simulink model "quadABLwind"  (R2018a)
settings: Solver=FixedStepAuto  StartTime=0.0  StopTime=50  FixedStep=.001  RelTol=1e-3  EnableMultiTasking=on
InitFcn:
  | parameters
model workspace: external: MAT-File C:\Users\Lab\Documents\MATLAB\projects\feedback_Ziegler_Quadrotor\parameters.mat (data not in the file)
values from neighbouring files (symbols this model uses):
  des_Position = zeros(10005/Ts + 1, 7)    [ABL_Quad_Traj.m]    (also in skyline_Quad_Traj.m = zeros(5005/Ts + 1, 7))
  wind_and_Max_Vel = abs([0, crosswind, maxVel])    [ABL_Quad_Traj.m]    (also in skyline_Quad_Traj.m)
  windECombined = [windE1; windE2; windE3; windE4; windE5; windE6; windE7]    [ABL_Quad_Traj.m]
  windNCombined = [windN1; windN2; windN3; windN4; windN5; windN6; windN7]    [ABL_Quad_Traj.m]
undefined symbols (not defined in the file or in its folder): DiscIntNeverNeededParam, P, starting_Point
libraries: simulink x1
settings Model: Creator=Lab  LastModifiedBy=lab
settings DataIOCC: ExternalInput=P
settings OptimizationCC: LifeSpan=inf
settings DebuggingCC: MultiTaskRateTransMsg=warning  SFUnexpectedBacktrackingDiag=warning  SFNoUnconditionalDefaultTransitionDiag=warning  SFExecutionAtInitializationDiag=none
settings CodeAppCC: StateflowObjectComments=on
settings GRTTargetCC: TargetLangStandard=C89/C90 (ANSI)  GeneratePreprocessorConditionals=Disable all
settings ConfigComp: CovMetricSettings=dw  CovHtmlReporting=on  CovSaveCumulativeToWorkspaceVar=on  CovSaveSingleToWorkspaceVar=on  CovExternalEMLEnable=off

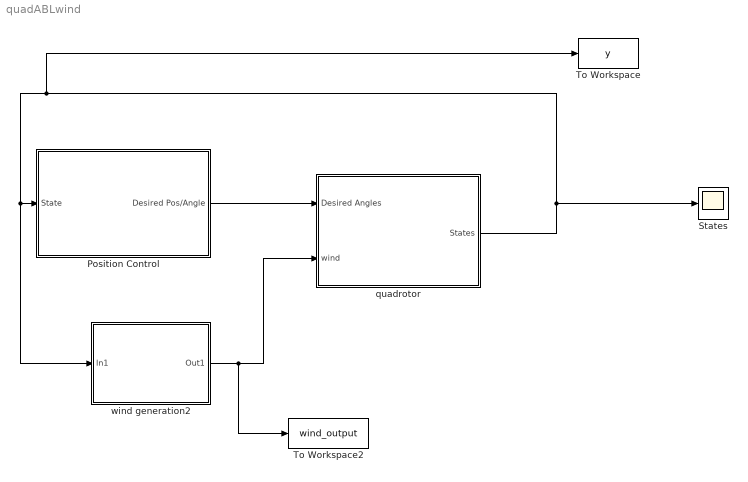
== system quadABLwind ==
  Position Control : Subsystem
  States : Scope
  To Workspace : ToWorkspace  VariableName=y  SaveFormat=Timeseries  SampleTime=-1
  To Workspace2 : ToWorkspace  VariableName=wind_output  SaveFormat=Timeseries  SampleTime=-1
  quadrotor : Subsystem
  wind generation2 : Subsystem
  wires:
  Position Control/1(Desired Pos/Angle) -> quadrotor/1(Desired Angles)
  wind generation2/1(Out1) -> To Workspace2/1, quadrotor/2(wind)
  quadrotor/1(States) -> To Workspace/1, wind generation2/1(In1), Position Control/1(State), States/1

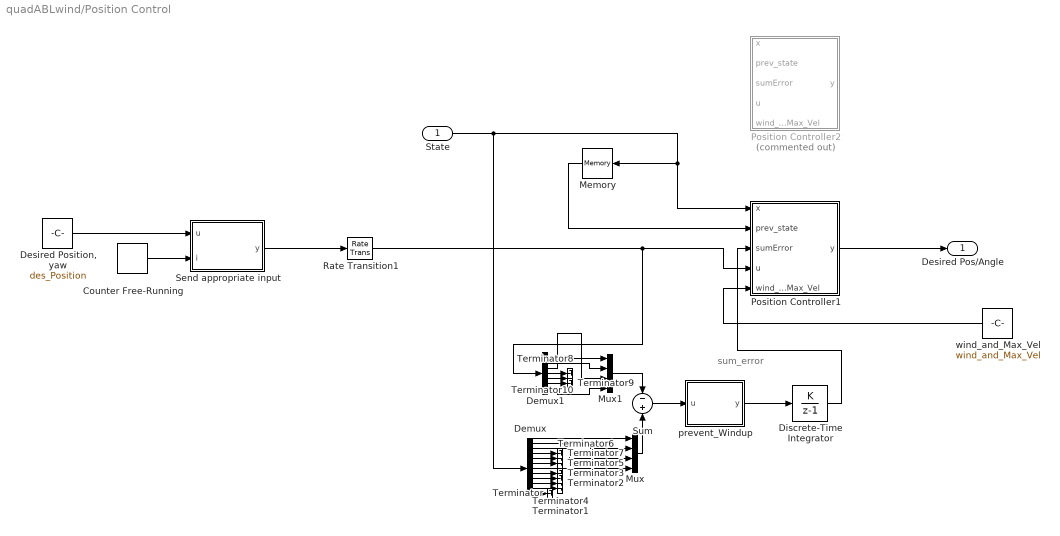
== system quadABLwind/Position Control ==
  note: sum_error
  State : Inport
  Counter Free-Running : simulink/Sources/Counter Free-Running  NumBits=32  tsamp=Ts
  Demux : Demux  Outputs=12
  Demux1 : Demux  Outputs=7
  "Desired Position, yaw" : Constant  Value=des_Position
  Discrete-Time Integrator : DiscreteIntegrator  IntegratorMethod=Accumulation: Forward Euler  gainval=1  SampleTime=-1  ICPrevOutput=DiscIntNeverNeededParam  ICPrevScaledInput=DiscIntNeverNeededParam
  Memory : Memory  InitialCondition=[0 0 0 0 0 0 0 0 0 0 0 0]
  Mux : Mux
  Mux1 : Mux
  Position Controller1 : MATLAB Function  TreatAsAtomicUnit=on  SystemSampleTime=P.Ts
  Position Controller2 : MATLAB Function  Commented=on  TreatAsAtomicUnit=on  SystemSampleTime=P.Ts
  Rate Transition1 : RateTransition  OutPortSampleTime=Tsd
  Send appropriate input : MATLAB Function  TreatAsAtomicUnit=on
  Sum : Sum  Inputs=-+
  Terminator{,1..10} (11 alike) : Terminator
  prevent_Windup : MATLAB Function  TreatAsAtomicUnit=on
  wind_and_Max_Vel : Constant  Value=wind_and_Max_Vel
  Desired Pos/Angle : Outport
  wires:
  Position Controller1/1(y) -> Desired Pos/Angle/1
  Mux/1 -> Sum/2
  Demux/1 -> Mux/1
  Demux/2 -> Mux/2
  Demux/3 -> Mux/3
  Memory/1 -> Position Controller1/2(prev_state)
  Sum/1 -> prevent_Windup/1(u)
  Demux/7 -> Mux/4
  "Desired Position, yaw"/1 -> Send appropriate input/1(u)
  Counter Free-Running/1 -> Send appropriate input/2(i)
  Send appropriate input/1(y) -> Rate Transition1/1
  State/1 -> Demux/1, Position Controller1/1(x), Memory/1
  Rate Transition1/1 -> Position Controller1/4(u), Demux1/1
  wind_and_Max_Vel/1 -> Position Controller1/5(wind_and_Max_Vel)
  Discrete-Time Integrator/1 -> Position Controller1/3(sumError)
  Demux1/1 -> Mux1/1
  Demux1/2 -> Mux1/2
  Demux1/3 -> Mux1/3
  Demux1/7 -> Mux1/4
  Mux1/1 -> Sum/1
  prevent_Windup/1(y) -> Discrete-Time Integrator/1
  Demux/12 -> Terminator/1
  Demux/8 -> Terminator3/1
  Demux/10 -> Terminator2/1
  Demux/11 -> Terminator1/1
  Demux/9 -> Terminator4/1
  Demux/6 -> Terminator5/1
  Demux/5 -> Terminator6/1
  Demux/4 -> Terminator7/1
  Demux1/4 -> Terminator8/1
  Demux1/6 -> Terminator9/1
  Demux1/5 -> Terminator10/1

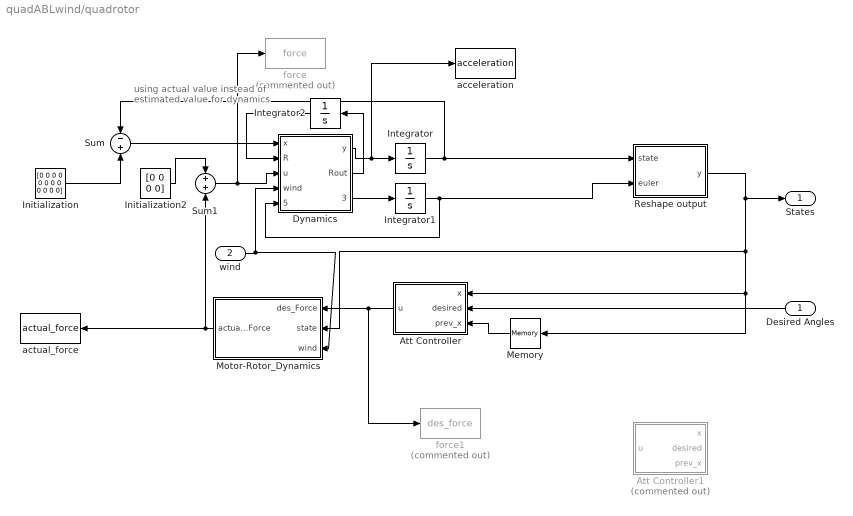
== system quadABLwind/quadrotor ==
  note: using actual value instead of estimated value for dynamics
  Desired Angles : Inport
  wind : Inport  Port=2
  Att Controller : MATLAB Function  TreatAsAtomicUnit=on
  Att Controller1 : MATLAB Function  Commented=on  TreatAsAtomicUnit=on
  Dynamics : MATLAB Function  TreatAsAtomicUnit=on  SystemSampleTime=P.Ts
  Initialization : Constant  Value=[0 0 0 0 0 0 0 0 0 0 0 0]
  Initialization2 : Constant  Value=[0 0 0 0]
  Integrator : Integrator
  Integrator1 : Integrator  InitialCondition=zeros(3,1)
  Integrator2 : Integrator  InitialCondition=eye(3)
  Memory : Memory  InitialCondition=[0 0 0 0 0 0 0 0 0 0 0 0]
  Motor-Rotor_Dynamics : Subsystem
  Reshape output : MATLAB Function  TreatAsAtomicUnit=on
  Sum : Sum  Inputs=-+
  Sum1 : Sum
  acceleration : ToWorkspace  VariableName=acceleration  SaveFormat=Timeseries  SampleTime=-1
  actual_force : ToWorkspace  VariableName=actual_force  SaveFormat=Timeseries  SampleTime=-1
  force : ToWorkspace  Commented=on  VariableName=force  SaveFormat=Timeseries  SampleTime=-1
  force1 : ToWorkspace  Commented=on  VariableName=des_force  SaveFormat=Timeseries  SampleTime=-1
  States : Outport
  wires:
  Sum1/1 -> Dynamics/3(u), force/1
  Dynamics/1(y) -> Integrator/1, acceleration/1
  Memory/1 -> Att Controller/3(prev_x)
  Sum/1 -> Dynamics/1(x)
  Integrator/1 -> Reshape output/1(state), Sum/1
  Initialization2/1 -> Sum1/1
  wind/1 -> Motor-Rotor_Dynamics/3(wind), Dynamics/4(wind)
  Initialization/1 -> Sum/2
  Desired Angles/1 -> Att Controller/2(desired)
  Att Controller/1(u) -> Motor-Rotor_Dynamics/1(des_Force), force1/1
  Motor-Rotor_Dynamics/1(actual_Force) -> actual_force/1, Sum1/2
  Dynamics/3(eulerout) -> Integrator1/1
  Integrator1/1 -> Dynamics/5(eulerin), Reshape output/2(euler)
  Dynamics/2(Rout) -> Integrator2/1
  Integrator2/1 -> Dynamics/2(R)
  Reshape output/1(y) -> Motor-Rotor_Dynamics/2(state), Memory/1, Att Controller/1(x), States/1

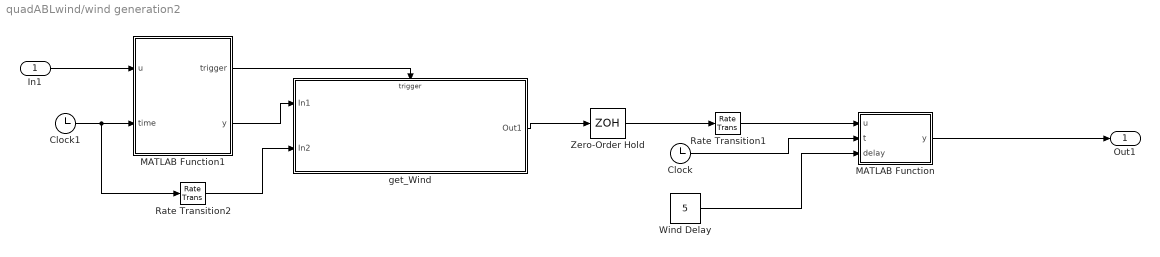
== system quadABLwind/wind generation2 ==
  In1 : Inport
  Clock : Clock
      settings: Decimation=3
  Clock1 : Clock
      settings: Decimation=3
  MATLAB Function : MATLAB Function  TreatAsAtomicUnit=on
  MATLAB Function1 : MATLAB Function  TreatAsAtomicUnit=on
  Rate Transition1 : RateTransition  OutPortSampleTime=Ts
  Rate Transition2 : RateTransition  OutPortSampleTime=0.1
  Wind Delay : Constant  Value=5
  Zero-Order Hold : ZeroOrderHold  SampleTime=0.1
  get_Wind : Subsystem
  Out1 : Outport
  wires:
  Rate Transition2/1 -> get_Wind/2(In2)
  MATLAB Function1/1(trigger) -> get_Wind/Trigger
  MATLAB Function1/2(y) -> get_Wind/1(In1)
  In1/1 -> MATLAB Function1/1(u)
  Clock1/1 -> MATLAB Function1/2(time), Rate Transition2/1
  get_Wind/1(Out1) -> Zero-Order Hold/1
  MATLAB Function/1(y) -> Out1/1
  Zero-Order Hold/1 -> Rate Transition1/1
  Rate Transition1/1 -> MATLAB Function/1(u)
  Wind Delay/1 -> MATLAB Function/3(delay)
  Clock/1 -> MATLAB Function/2(t)

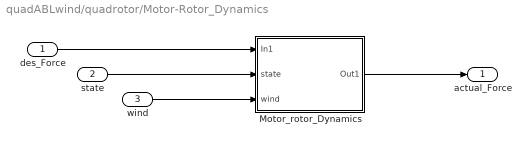
== system quadABLwind/quadrotor/Motor-Rotor_Dynamics ==
  des_Force : Inport
  state : Inport  Port=2
  wind : Inport  Port=3
  Motor_rotor_Dynamics : Subsystem
  actual_Force : Outport
  wires:
  des_Force/1 -> Motor_rotor_Dynamics/1(In1)
  state/1 -> Motor_rotor_Dynamics/2(state)
  wind/1 -> Motor_rotor_Dynamics/3(wind)
  Motor_rotor_Dynamics/1(Out1) -> actual_Force/1

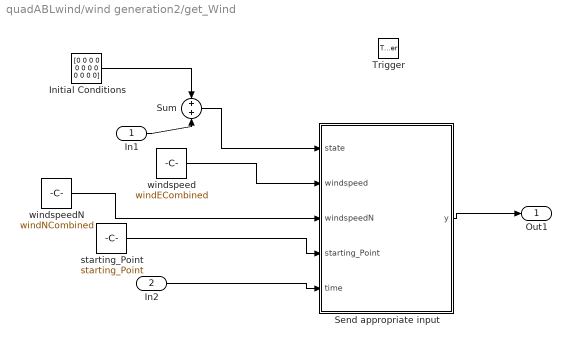
== system quadABLwind/wind generation2/get_Wind ==
  In1 : Inport
  In2 : Inport  Port=2
  Trigger : TriggerPort  VariantControl=Variant  PortDimensions=1
  Initial Conditions : Constant  Value=[0 0 0 0 0 0 0 0 0 0 0 0]
  Send appropriate input : MATLAB Function  TreatAsAtomicUnit=on
  Sum : Sum
  starting_Point : Constant  Value=starting_Point
  windspeed : Constant  Value=windECombined
  windspeedN : Constant  Value=windNCombined
  Out1 : Outport
  wires:
  windspeedN/1 -> Send appropriate input/3(windspeedN)
  starting_Point/1 -> Send appropriate input/4(starting_Point)
  In2/1 -> Send appropriate input/5(time)
  Send appropriate input/1(y) -> Out1/1
  In1/1 -> Sum/2
  windspeed/1 -> Send appropriate input/2(windspeed)
  Sum/1 -> Send appropriate input/1(state)
  Initial Conditions/1 -> Sum/1

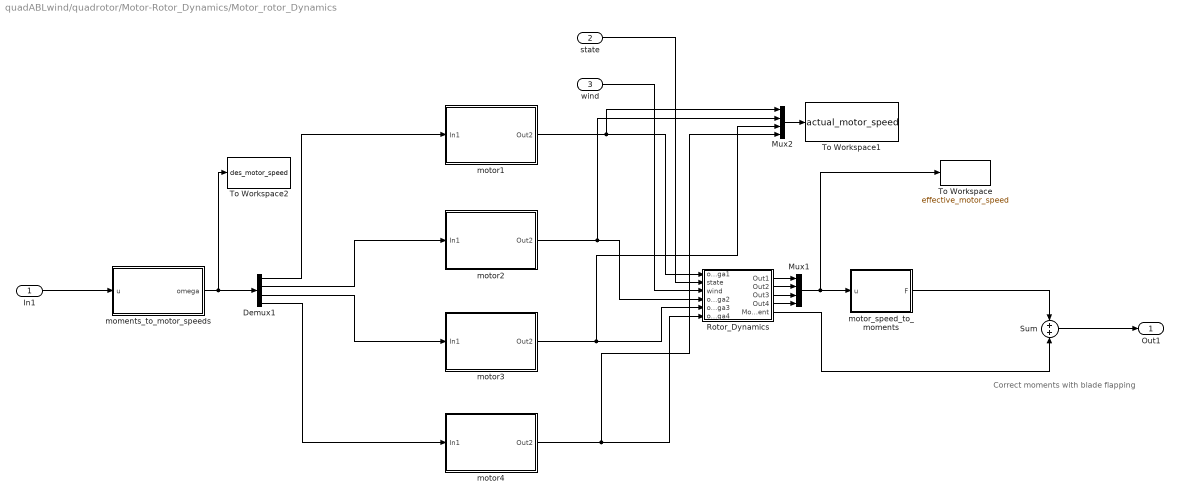
== system quadABLwind/quadrotor/Motor-Rotor_Dynamics/Motor_rotor_Dynamics ==
  note: Correct moments with blade flapping
  In1 : Inport
  state : Inport  Port=2
  wind : Inport  Port=3
  Demux1 : Demux
  Mux1 : Mux
  Mux2 : Mux
  Rotor_Dynamics : Subsystem
  Sum : Sum
  To Workspace : ToWorkspace  VariableName=effective_motor_speed  SaveFormat=Timeseries  SampleTime=-1
      settings: Save2DSignal=2-D array (concatenate along first dimension)
  To Workspace1 : ToWorkspace  VariableName=actual_motor_speed  SaveFormat=Timeseries  SampleTime=-1
      settings: Save2DSignal=2-D array (concatenate along first dimension)
  To Workspace2 : ToWorkspace  VariableName=des_motor_speed  SaveFormat=Timeseries  SampleTime=-1
      settings: Save2DSignal=2-D array (concatenate along first dimension)
  moments_to_motor_speeds : MATLAB Function  TreatAsAtomicUnit=on
  motor1 : Subsystem
  motor2 : Subsystem
  motor3 : Subsystem
  motor4 : Subsystem
  motor_speed_to_moments : MATLAB Function  TreatAsAtomicUnit=on
  Out1 : Outport
  wires:
  In1/1 -> moments_to_motor_speeds/1(u)
  motor_speed_to_moments/1(F) -> Sum/1
  Demux1/1 -> motor1/1(In1)
  moments_to_motor_speeds/1(omega) -> To Workspace2/1, Demux1/1
  Demux1/2 -> motor2/1(In1)
  motor4/1(Out2) -> Mux2/4, Rotor_Dynamics/6(omega4)
  motor2/1(Out2) -> Mux2/2, Rotor_Dynamics/4(omega2)
  Demux1/3 -> motor3/1(In1)
  Demux1/4 -> motor4/1(In1)
  motor3/1(Out2) -> Mux2/3, Rotor_Dynamics/5(omega3)
  Mux1/1 -> To Workspace/1, motor_speed_to_moments/1(u)
  wind/1 -> Rotor_Dynamics/3(wind)
  state/1 -> Rotor_Dynamics/2(state)
  Rotor_Dynamics/2(Out2) -> Mux1/2
  Rotor_Dynamics/3(Out3) -> Mux1/3
  Rotor_Dynamics/4(Out4) -> Mux1/4
  Rotor_Dynamics/1(Out1) -> Mux1/1
  Rotor_Dynamics/5(Moment) -> Sum/2
  Sum/1 -> Out1/1
  motor1/1(Out2) -> Mux2/1, Rotor_Dynamics/1(omega1)
  Mux2/1 -> To Workspace1/1

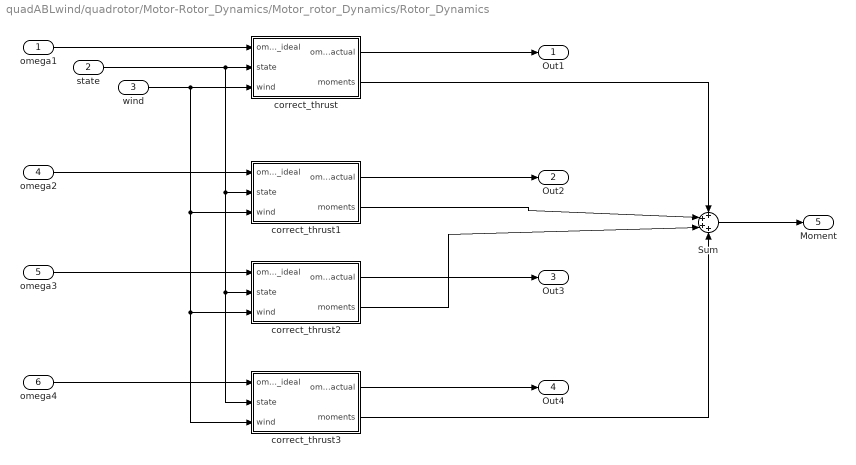
== system quadABLwind/quadrotor/Motor-Rotor_Dynamics/Motor_rotor_Dynamics/Rotor_Dynamics ==
  omega1 : Inport
  state : Inport  Port=2
  wind : Inport  Port=3
  omega2 : Inport  Port=4
  omega3 : Inport  Port=5
  omega4 : Inport  Port=6
  Sum : Sum  Inputs=++++
  correct_thrust : MATLAB Function  TreatAsAtomicUnit=on
  correct_thrust1 : MATLAB Function  TreatAsAtomicUnit=on
  correct_thrust2 : MATLAB Function  TreatAsAtomicUnit=on
  correct_thrust3 : MATLAB Function  TreatAsAtomicUnit=on
  Out1 : Outport
  Out2 : Outport  Port=2
  Out3 : Outport  Port=3
  Out4 : Outport  Port=4
  Moment : Outport  Port=5
  wires:
  correct_thrust/1(omega_actual) -> Out1/1
  omega1/1 -> correct_thrust/1(omega_ideal)
  state/1 -> correct_thrust1/2(state), correct_thrust3/2(state), correct_thrust2/2(state), correct_thrust/2(state)
  wind/1 -> correct_thrust1/3(wind), correct_thrust3/3(wind), correct_thrust2/3(wind), correct_thrust/3(wind)
  omega2/1 -> correct_thrust1/1(omega_ideal)
  omega3/1 -> correct_thrust2/1(omega_ideal)
  omega4/1 -> correct_thrust3/1(omega_ideal)
  correct_thrust3/1(omega_actual) -> Out4/1
  correct_thrust2/1(omega_actual) -> Out3/1
  correct_thrust1/1(omega_actual) -> Out2/1
  correct_thrust/2(moments) -> Sum/1
  correct_thrust1/2(moments) -> Sum/2
  correct_thrust2/2(moments) -> Sum/3
  correct_thrust3/2(moments) -> Sum/4
  Sum/1 -> Moment/1

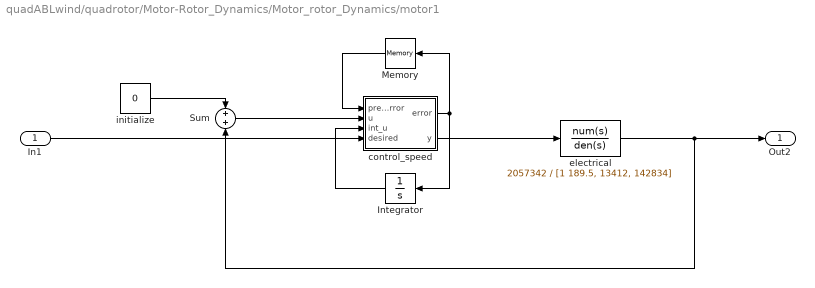
== system quadABLwind/quadrotor/Motor-Rotor_Dynamics/Motor_rotor_Dynamics/motor1 ==
  In1 : Inport
  Integrator : Integrator
  Memory : Memory  InitialCondition=[0]
  Sum : Sum
  control_speed : MATLAB Function  TreatAsAtomicUnit=on
  electrical : TransferFcn  Numerator=2057342  Denominator=[1 189.5, 13412, 142834]
  initialize : Constant  Value=0
  Out2 : Outport
  wires:
  control_speed/2(y) -> electrical/1
  In1/1 -> control_speed/4(desired)
  electrical/1 -> Sum/2, Out2/1
  Sum/1 -> control_speed/2(u)
  Memory/1 -> control_speed/1(prev_error)
  Integrator/1 -> control_speed/3(int_u)
  initialize/1 -> Sum/1
  control_speed/1(error) -> Integrator/1, Memory/1

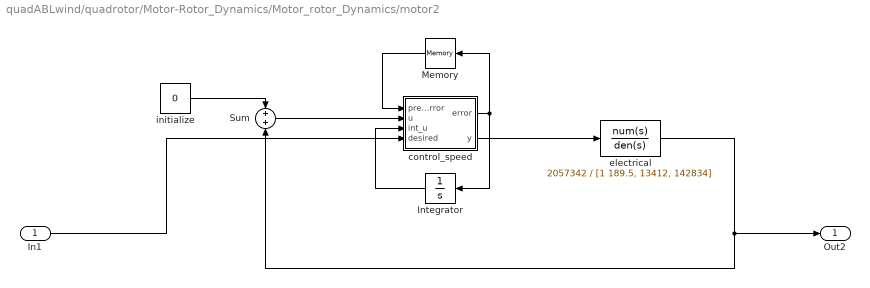
== system quadABLwind/quadrotor/Motor-Rotor_Dynamics/Motor_rotor_Dynamics/motor2 ==
  In1 : Inport
  Integrator : Integrator
  Memory : Memory  InitialCondition=[0]
  Sum : Sum
  control_speed : MATLAB Function  TreatAsAtomicUnit=on
  electrical : TransferFcn  Numerator=2057342  Denominator=[1 189.5, 13412, 142834]
  initialize : Constant  Value=0
  Out2 : Outport
  wires:
  control_speed/1(error) -> Memory/1, Integrator/1
  initialize/1 -> Sum/1
  Integrator/1 -> control_speed/3(int_u)
  Memory/1 -> control_speed/1(prev_error)
  Sum/1 -> control_speed/2(u)
  electrical/1 -> Sum/2, Out2/1
  In1/1 -> control_speed/4(desired)
  control_speed/2(y) -> electrical/1

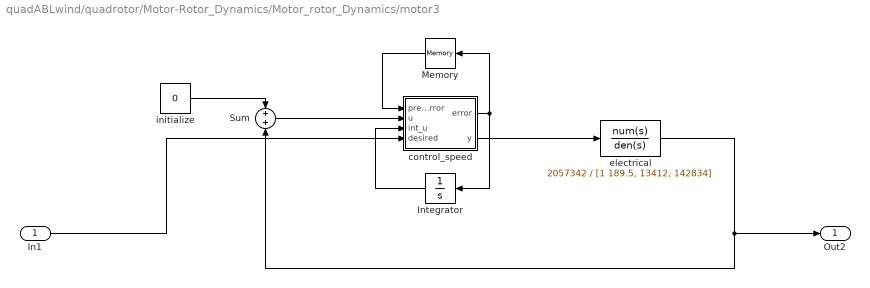
== system quadABLwind/quadrotor/Motor-Rotor_Dynamics/Motor_rotor_Dynamics/motor3 ==
  In1 : Inport
  Integrator : Integrator
  Memory : Memory  InitialCondition=[0]
  Sum : Sum
  control_speed : MATLAB Function  TreatAsAtomicUnit=on
  electrical : TransferFcn  Numerator=2057342  Denominator=[1 189.5, 13412, 142834]
  initialize : Constant  Value=0
  Out2 : Outport
  wires:
  control_speed/2(y) -> electrical/1
  In1/1 -> control_speed/4(desired)
  electrical/1 -> Out2/1, Sum/2
  Sum/1 -> control_speed/2(u)
  Memory/1 -> control_speed/1(prev_error)
  Integrator/1 -> control_speed/3(int_u)
  initialize/1 -> Sum/1
  control_speed/1(error) -> Integrator/1, Memory/1

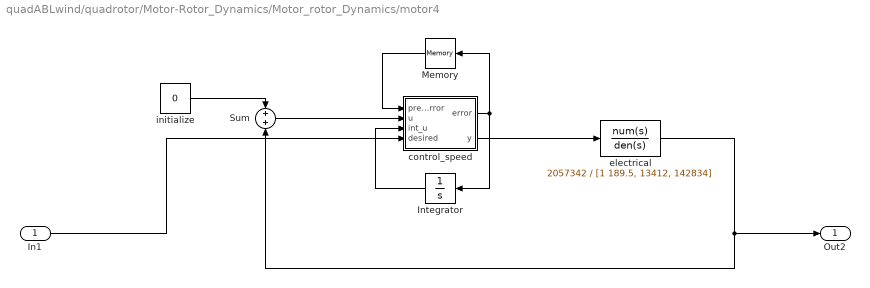
== system quadABLwind/quadrotor/Motor-Rotor_Dynamics/Motor_rotor_Dynamics/motor4 ==
  In1 : Inport
  Integrator : Integrator
  Memory : Memory  InitialCondition=[0]
  Sum : Sum
  control_speed : MATLAB Function  TreatAsAtomicUnit=on
  electrical : TransferFcn  Numerator=2057342  Denominator=[1 189.5, 13412, 142834]
  initialize : Constant  Value=0
  Out2 : Outport
  wires:
  control_speed/1(error) -> Memory/1, Integrator/1
  initialize/1 -> Sum/1
  Integrator/1 -> control_speed/3(int_u)
  Memory/1 -> control_speed/1(prev_error)
  Sum/1 -> control_speed/2(u)
  electrical/1 -> Sum/2, Out2/1
  In1/1 -> control_speed/4(desired)
  control_speed/2(y) -> electrical/1

== matlab function quadABLwind/quadrotor/Att Controller ==
  data: x input; u output; desired input; prev_x input; P parameter
function u = fcn(x, desired, prev_x, P)
%#codegen
% Reference: A Simple Attitude Control of Quadrotor Helicopter Based on
%Ziegler-Nichols Rules for Tuning PD Parameters

%ZeFang He and Long Zhao

u = zeros(4,1);
%timestep size
Ts = P.Ts;

L = P.L;  Ix = P.Ix;  Iy = P.Iy;  Iz = P.Iz; m = P.m; g = P.g;
b1 = 1/Ix;
b2 = 1/Iy;
b3 = 1/Iz;

a1 = (Iy-Iz)/Ix;
a3 = (Iz-Ix)/Iy;
a5 = (Ix-Iy)/Iz;

K2 = P.K2;
K3 = P.K3;
K4 = P.K4;

Kp2 = P.Kp2;
Kp3 = P.Kp3;
Kp4 = P.Kp4;

Kd2 = P.Kd2;
Kd3 = P.Kd3;
Kd4 = P.Kd4;


err2 = (desired(7) - x(7));
err3 = (desired(8) - x(8));
err4 = (desired(9) - x(9));
prev_err2 = (desired(7) - prev_x(7));
prev_err3 = (desired(8) - prev_x(8));
prev_err4 = (desired(9) - prev_x(9));

err_tot = [err2;err3;err4];
prev_err_tot = [prev_err2;prev_err3;prev_err4];

u(1) = (m*g + desired(3)*m)/(cos(x(7)) * cos(x(8)));
% u(2) = 1/b1*(K2*x(10)-a1*x(11)*x(12)) + Kp2*err2 + Kd2*(err2-prev_err2)/Ts;
% u(3) = 1/b2*(K3*x(11)-a3*x(10)*x(12)) + Kp3*err3 + Kd3*(err3-prev_err3)/Ts;
% u(4) = 1/b3*(K4*x(12)-a5*x(10)*x(11)) + Kp4*err4 + Kd4*(err4-prev_err4)/Ts;
u(2:4) = P.I*(K2*x(10:12)) + cross(x(10:12),P.I*x(10:12)) + Kp2*err_tot + Kd2*(err_tot-prev_err_tot)/Ts;

% u(1) = (m*g + desired(3)*m)/(cos(euler(1)) * cos(euler(2)));
% u(2) = 1/b1*(K2*x(10)-a1*x(11)*x(12)) + Kp2*err2 + Kd2*(err2-prev_err2)/Ts;
% u(3) = 1/b2*(K3*x(11)-a3*x(10)*x(12)) + Kp3*err3 + Kd3*(err3-prev_err3)/Ts;
% u(4) = 1/b3*(K4*x(12)-a5*x(10)*x(11)) + Kp4*err4 + Kd4*(err4-prev_err4)/Ts;

== matlab function quadABLwind/Position Control/Position Controller1 ==
  data: x input; prev_state input; sumError input; u input; y output; wind_and_Max_Vel input; P parameter
function y  = fcn(x, prev_state, sumError, u, wind_and_Max_Vel, P)
%#codegen
%PID controller tuned by hand
phi=x(7);
theta = x(8);
psi = x(9);

x_error1 = (u(1) + x(1));
y_error1 = (u(2) + x(2));

% R = [cos(theta)*cos(phi)-cos(psi)*sin(phi)*sin(psi), -cos(psi)*sin(phi),...
%     cos(phi)*sin(theta)+cos(theta)*sin(phi)*sin(psi); ...
%     cos(theta)*sin(phi)+cos(phi)*sin(theta)*sin(psi), cos(phi)*cos(psi),...
%     sin(theta)*sin(phi)-cos(theta)*cos(phi)*sin(psi);...
%     -cos(psi)*sin(theta), sin(psi), cos(theta)*cos(psi)];

R = [cos(psi), sin(psi), 0; -sin(psi), cos(psi), 0; 0, 0, 1];


x(1:3) = R*x(1:3);
u(1:3) = (R*u(1:3)')';
prev_state(1:3) = R*prev_state(1:3);
sumError(1:3) = R*sumError(1:3);

% u = xyz, yaw
y = zeros(12,1);
Ts = P.Ts;
g = P.g;
m = P.m;

Cd=zeros(3,1);
Cd(1:3) = P.Cd1 + 0.9*exp(-0.6*(norm(wind_and_Max_Vel+x(4))-2));
for i=1:3
    if Cd(i) > 1.1
        Cd(i) = 1.1;
    end
end 

%control 7,8,9 for roll, pitch, yaw angles
u = -u;


x_error = (u(1) + x(1));
y_error = (u(2) + x(2));
z_error = u(3) + x(3);


%previous errors
px_error = (u(1) + prev_state(1));
py_error = (u(2) + prev_state(2));
pz_error = u(3) + prev_state(3);


vx_error = (u(4) + x(4));
vy_error = (u(5) + x(5));


kp = P.kp;
kd = P.kd;
%ki currently set to zero.  Using PD control
ki = P.ki;


%PID controller for y, x, and yaw.  Sends roll/pitch angles to attitude
%controller
y(7) = (kp*y_error + kd*vy_error) + ki*sumError(2);
y(8) = (kp*x_error + kd*vx_error) + ki*sumError(1);


y(9) = -u(7);

k2 = P.k2;
kd2 = P.kd2;
ki2 = P.ki2;
%altitude control
y(3) = k2*z_error + kd2*(z_error - pz_error)/Ts + ki2*sumError(3);

% if abs(y(3))>6
%     y(3)=sign(y(3))*6;
% end

%ensure that the norm of velocity is correct since the pitch is hardcoded
if abs(wind_and_Max_Vel(3)) < abs(x(4))
    wind_and_Max_Vel(3) = x(4);
end

mag_V = wind_and_Max_Vel(1:2) + wind_and_Max_Vel(3:4);
mag_Combined = norm(mag_V); %airspeed magnitude

F_w = zeros(2,1);
F_w(1) = Cd(1) * mag_Combined^2;
F_w(2) = Cd(2) * mag_Combined^2;

%roll, pitch angles determined by desired y, x velocities and windspeed
max_Angle = zeros(1,2);
max_Angle(1) = 0.8;%atan2(F_w(2) * mag_V(2), m*g*mag_Combined);
max_Angle(2) = 0.8;%0.535;

if max_Angle(1) > 0.8
    max_Angle(1) = 0.8;
end

if y(7) > max_Angle(1)
    y(7) = max_Angle(1);

elseif y(7) < -max_Angle(1)
    y(7) = -max_Angle(1);
end
if y(8) > max_Angle(2)
    y(8) = max_Angle(2);
elseif y(8) < -max_Angle(2)
    y(8) = -max_Angle(2);
end

%set maximum total angle to 0.8 radians
% angleNorm = norm(y(7:8));
% if angleNorm > 0.8
%     y(7) = y(7)/(angleNorm)*(0.8);
%     y(8) = y(8)/(angleNorm)*(0.8);
% end

end

== matlab function quadABLwind/wind generation2/MATLAB Function ==
  data: u input; t input; y output; delay input
function y = fcn(u, t, delay)
%#codegen

if delay - t > 0% || delay-t < -1
    y = zeros(size(u));% + 10*randn(size(u));
else
    y = u;% + 10*randn(size(u));%[0; 10*randn(1); 0];
end

== matlab function quadABLwind/quadrotor/Motor-Rotor_Dynamics/Motor_rotor_Dynamics/Rotor_Dynamics/correct_thrust ==
  data: omega_ideal input; state input; wind input; omega_actual output; P parameter; moments output
function [omega_actual, moments] = fcn(omega_ideal, state, wind, P)
%from "Dynamic Control of Autonomous Quadrotor Flight in an Estimated Wind
%Field," by Sydney, Smyth, and Paley
omega_actual=omega_ideal;

%ensure nonzero rotor speed
if omega_ideal<0
    omega_ideal=0;
end

T_ideal = P.k_t*omega_ideal.^2;

phi = state(7);
theta = state(8);
psi = state(9);

%induced velocity of air
v_h = sqrt(T_ideal/(2*P.rho*pi*P.R^2));

% rotation from inertial frame to body frame
R = [1, 0, 0;0, cos(phi), sin(phi);0, -sin(phi), cos(phi)]*[cos(theta),...
    0, -sin(theta);0, 1, 0;sin(theta), 0, cos(theta)]*[cos(psi),...
    sin(psi), 0;-sin(psi), cos(psi), 0;0, 0, 1];

%find u, v, w (airspeeds on rotor in body frame)
air_vel = R*(state(4:6)+wind);
air_vel(3) = -air_vel(3);

%model blade flapping when airspeed > 1 m/s
if sqrt(air_vel(1)^2+air_vel(2)^2)>.1
    alpha = P.kf_rotor*sqrt(air_vel(1)^2+air_vel(2)^2);
    u_bar = air_vel(1)/sqrt(air_vel(1)^2+air_vel(2)^2);
    v_bar = air_vel(2)/sqrt(air_vel(1)^2+air_vel(2)^2);

    T_flap_vec = T_ideal*[u_bar*sin(alpha), v_bar*sin(alpha), cos(alpha)];
    T_flap = T_flap_vec(3);
else
    T_flap_vec = [0, 0, T_ideal];
    T_flap = T_ideal;
end



if air_vel(3)>2*abs(v_h)
    
    p = [1 2*air_vel(3) (air_vel(1)^2+air_vel(2)^2+air_vel(3)^2) 0 -v_h^4];
    vi = max(real(roots(p)));

    if norm(air_vel)<=0.5
        vi = v_h;
    end

    T_actual = T_flap*vi/(vi+air_vel(3));
else
    T_actual = T_flap;
end

omega_actual = sqrt(T_actual/P.k_t);
moments = [0 T_flap_vec(2:-1:1) 0];

if omega_actual>1000
    omega_actual=1000;
end


end

== matlab function quadABLwind/quadrotor/Motor-Rotor_Dynamics/Motor_rotor_Dynamics/Rotor_Dynamics/correct_thrust1 ==
  data: omega_ideal input; state input; wind input; omega_actual output; P parameter; moments output
function [omega_actual, moments] = fcn(omega_ideal, state, wind, P)
%from "Dynamic Control of Autonomous Quadrotor Flight in an Estimated Wind
%Field," by Sydney, Smyth, and Paley
omega_actual=omega_ideal;

%ensure nonzero rotor speed
if omega_ideal<0
    omega_ideal=0;
end

T_ideal = P.k_t*omega_ideal.^2;

phi = state(7);
theta = state(8);
psi = state(9);

%induced velocity of air
v_h = sqrt(T_ideal/(2*P.rho*pi*P.R^2));

% rotation from inertial frame to body frame
R = [1, 0, 0;0, cos(phi), sin(phi);0, -sin(phi), cos(phi)]*[cos(theta),...
    0, -sin(theta);0, 1, 0;sin(theta), 0, cos(theta)]*[cos(psi),...
    sin(psi), 0;-sin(psi), cos(psi), 0;0, 0, 1];

%find u, v, w (airspeeds on rotor in body frame)
air_vel = R*(state(4:6)+wind);
air_vel(3) = -air_vel(3);

%model blade flapping when airspeed > 1 m/s
if sqrt(air_vel(1)^2+air_vel(2)^2)>.1
    alpha = P.kf_rotor*sqrt(air_vel(1)^2+air_vel(2)^2);
    u_bar = air_vel(1)/sqrt(air_vel(1)^2+air_vel(2)^2);
    v_bar = air_vel(2)/sqrt(air_vel(1)^2+air_vel(2)^2);

    T_flap_vec = T_ideal*[u_bar*sin(alpha), v_bar*sin(alpha), cos(alpha)];
    T_flap = T_flap_vec(3);
else
    T_flap_vec = [0, 0, T_ideal];
    T_flap = T_ideal;
end



if air_vel(3)>2*abs(v_h)
    
    p = [1 2*air_vel(3) (air_vel(1)^2+air_vel(2)^2+air_vel(3)^2) 0 -v_h^4];
    vi = max(real(roots(p)));

    if norm(air_vel)<=0.5
        vi = v_h;
    end

    T_actual = T_flap*vi/(vi+air_vel(3));
else
    T_actual = T_flap;
end

omega_actual = sqrt(T_actual/P.k_t);
moments = [0 T_flap_vec(2:-1:1) 0];

if omega_actual>1000
    omega_actual=1000;
end


end

== matlab function quadABLwind/quadrotor/Dynamics ==
  data: x input size=[12,1]; R input; u input; y output; Rout output; wind input size=[3,1]; eulerin input; P parameter; eulerout output size=[3 1]
function [y, Rout, eulerout] = fcn(x, R, u, wind, eulerin, P)
%#codegen
%References: Quadrotor Dynamics and Control Rev 0.1
%Randal Beard

%A Simple Attitude Control of Quadrotor Helicopter Based on
%Ziegler-Nichols Rules for Tuning PD Parameters
%ZeFang He and Long Zhao

m = P.m;
g = P.g;
Ix = P.Ix;
Iy = P.Iy;
Iz = P.Iz;
L = P.L;



Cd = zeros(3,1);
Cd(1:3) = P.Cd1 + 0.9*exp(-0.6*(norm(wind(1:3)+x(4:6))-2));


for i=1:3
    if Cd(i) > 1.1
        Cd(i) = 1.1;
    end
end

y = x;

%Calculate drag force on quadrotor
mag_V = wind + x(4:6);

mag_Combined = norm(mag_V); %airspeed magnitude
force = Cd * mag_Combined^2;

Fw = zeros(3,1);
if mag_Combined ~= 0
    Fw = diag(mag_V/mag_Combined) * force;
else
    Fw(:) = 0;
end


y(1) = -x(4);
y(2) = -x(5);
y(3) = -x(6);
y(4) = (u(1))/m*(cos(x(7))*sin(x(8))*cos(x(9)) +...
    sin(x(7))*sin(x(9))) + Fw(1)/m;
y(5) = -(u(1))/m*(+cos(x(7))*sin(x(8))*sin(x(9)) -...
    sin(x(7))*cos(x(9))) + Fw(2)/m;
y(6) = g - (u(1))/m*(cos(x(7)) * cos(x(8))) + Fw(3);

%y(4:6) = (P.g*P.e3 - u(1)*R*P.e3/P.m + Fw);


%p, q, r
y(7) = -x(10);
y(8) = -x(11);
y(9) = -x(12);
% y(10) = x(11)*x(12)*(Iy-Iz)/Ix + u(2)/Ix;
% y(11) = x(10)*x(12)*(Iz-Ix)/Iy + u(3)/Iy;
% y(12) = x(10)*x(11)*(Ix - Iy)/Iz + u(4)/Iz;
y(10:12) = inv(P.I)*u(2:4) - inv(P.I)*cross(y(10:12), P.I*y(10:12));

omega_hat = [0 -y(9) y(8); y(9) 0 -y(7); -y(8) y(7) 0];
Rout = cross(R,omega_hat);

%roll, pitch, yaw: phi, theta, psi
phi = eulerin(1);
theta = eulerin(2);
psi = eulerin(3);
Reuler = [1 sin(phi)*tan(theta) cos(phi)*tan(theta);
          0 cos(phi) -sin(phi);
          0 sin(phi)/cos(theta) cos(phi)/cos(theta)];

eulerout = Reuler*y(7:9);

== matlab function quadABLwind/quadrotor/Motor-Rotor_Dynamics/Motor_rotor_Dynamics/Rotor_Dynamics/correct_thrust2 ==
  data: omega_ideal input; state input; wind input; omega_actual output; P parameter; moments output
function [omega_actual, moments] = fcn(omega_ideal, state, wind, P)
%from "Dynamic Control of Autonomous Quadrotor Flight in an Estimated Wind
%Field," by Sydney, Smyth, and Paley
omega_actual=omega_ideal;

%ensure nonzero rotor speed
if omega_ideal<0
    omega_ideal=0;
end

T_ideal = P.k_t*omega_ideal.^2;

phi = state(7);
theta = state(8);
psi = state(9);

%induced velocity of air
v_h = sqrt(T_ideal/(2*P.rho*pi*P.R^2));

% rotation from inertial frame to body frame
R = [1, 0, 0;0, cos(phi), sin(phi);0, -sin(phi), cos(phi)]*[cos(theta),...
    0, -sin(theta);0, 1, 0;sin(theta), 0, cos(theta)]*[cos(psi),...
    sin(psi), 0;-sin(psi), cos(psi), 0;0, 0, 1];

%find u, v, w (airspeeds on rotor in body frame)
air_vel = R*(state(4:6)+wind);
air_vel(3) = -air_vel(3);

%model blade flapping when airspeed > 1 m/s
if sqrt(air_vel(1)^2+air_vel(2)^2)>.1
    alpha = P.kf_rotor*sqrt(air_vel(1)^2+air_vel(2)^2);
    u_bar = air_vel(1)/sqrt(air_vel(1)^2+air_vel(2)^2);
    v_bar = air_vel(2)/sqrt(air_vel(1)^2+air_vel(2)^2);

    T_flap_vec = T_ideal*[u_bar*sin(alpha), v_bar*sin(alpha), cos(alpha)];
    T_flap = T_flap_vec(3);
else
    T_flap_vec = [0, 0, T_ideal];
    T_flap = T_ideal;
end



if air_vel(3)>2*abs(v_h)
    
    p = [1 2*air_vel(3) (air_vel(1)^2+air_vel(2)^2+air_vel(3)^2) 0 -v_h^4];
    vi = max(real(roots(p)));

    if norm(air_vel)<=0.5
        vi = v_h;
    end

    T_actual = T_flap*vi/(vi+air_vel(3));
else
    T_actual = T_flap;
end

omega_actual = sqrt(T_actual/P.k_t);
moments = [0 T_flap_vec(2:-1:1) 0];

if omega_actual>1000
    omega_actual=1000;
end


end

== matlab function quadABLwind/quadrotor/Motor-Rotor_Dynamics/Motor_rotor_Dynamics/Rotor_Dynamics/correct_thrust3 ==
  data: omega_ideal input; state input; wind input; omega_actual output; P parameter; moments output
function [omega_actual, moments] = fcn(omega_ideal, state, wind, P)
%from "Dynamic Control of Autonomous Quadrotor Flight in an Estimated Wind
%Field," by Sydney, Smyth, and Paley
omega_actual=omega_ideal;

%ensure nonzero rotor speed
if omega_ideal<0
    omega_ideal=0;
end

T_ideal = P.k_t*omega_ideal.^2;

phi = state(7);
theta = state(8);
psi = state(9);

%induced velocity of air
v_h = sqrt(T_ideal/(2*P.rho*pi*P.R^2));

% rotation from inertial frame to body frame
R = [1, 0, 0;0, cos(phi), sin(phi);0, -sin(phi), cos(phi)]*[cos(theta),...
    0, -sin(theta);0, 1, 0;sin(theta), 0, cos(theta)]*[cos(psi),...
    sin(psi), 0;-sin(psi), cos(psi), 0;0, 0, 1];

%find u, v, w (airspeeds on rotor in body frame)
air_vel = R*(state(4:6)+wind);
air_vel(3) = -air_vel(3);

%model blade flapping when airspeed > 1 m/s
if sqrt(air_vel(1)^2+air_vel(2)^2)>.1
    alpha = P.kf_rotor*sqrt(air_vel(1)^2+air_vel(2)^2);
    u_bar = air_vel(1)/sqrt(air_vel(1)^2+air_vel(2)^2);
    v_bar = air_vel(2)/sqrt(air_vel(1)^2+air_vel(2)^2);

    T_flap_vec = T_ideal*[u_bar*sin(alpha), v_bar*sin(alpha), cos(alpha)];
    T_flap = T_flap_vec(3);
else
    T_flap_vec = [0, 0, T_ideal];
    T_flap = T_ideal;
end



if air_vel(3)>2*abs(v_h)
    
    p = [1 2*air_vel(3) (air_vel(1)^2+air_vel(2)^2+air_vel(3)^2) 0 -v_h^4];
    vi = max(real(roots(p)));

    if norm(air_vel)<=0.5
        vi = v_h;
    end

    T_actual = T_flap*vi/(vi+air_vel(3));
else
    T_actual = T_flap;
end

omega_actual = sqrt(T_actual/P.k_t);
moments = [0 T_flap_vec(2:-1:1) 0];

if omega_actual>1000
    omega_actual=1000;
end


end

== matlab function quadABLwind/Position Control/Send appropriate input ==
  data: u input; y output; i input
function y = fcn(u, i)
%#codegen

y = u(i+1,:);

== matlab function quadABLwind/quadrotor/Motor-Rotor_Dynamics/Motor_rotor_Dynamics/motor2/control_speed ==
  data: error output; prev_error input; u input; y output; int_u input; desired input; P parameter
function [error, y] = fcn(prev_error, u, int_u, desired, P)

%y = u;
if desired > 1000
    desired = 1000;
end

error = (desired-u);

Ts = P.Ts;

% kd = .2;
% kp = 10;
% ki = 5;

% kd = 0.05;
% kp = 1;
% ki = 1;

kd = P.kd_motor;
kp = P.kp_motor;
ki = P.ki_motor;

edot = ((error)-(prev_error))/Ts;

y = (kd*edot + kp*(error) + ki*int_u);

%saturate pwm at 2000
if abs(y) > 2000
    y = sign(y)*2000;
end

== matlab function quadABLwind/Position Control/prevent_Windup ==
  data: u input; y output
function y = fcn(u)
%#codegen
y=u;
%y(1)=0;

for i=1:4
    
    if abs(u(i))>20
        y(i)=0;
    end
end

== matlab function quadABLwind/quadrotor/Motor-Rotor_Dynamics/Motor_rotor_Dynamics/motor3/control_speed ==
  data: error output; prev_error input; u input; y output; int_u input; desired input; P parameter
function [error, y] = fcn(prev_error, u, int_u, desired, P)

%y = u;
if desired > 1000
    desired = 1000;
end

error = (desired-u);

Ts = P.Ts;

% kd = .2;
% kp = 10;
% ki = 5;

% kd = 0.05;
% kp = 1;
% ki = 1;

kd = P.kd_motor;
kp = P.kp_motor;
ki = P.ki_motor;

edot = ((error)-(prev_error))/Ts;

y = (kd*edot + kp*(error) + ki*int_u);

%saturate pwm at 2000
if abs(y) > 2000
    y = sign(y)*2000;
end

== matlab function quadABLwind/quadrotor/Motor-Rotor_Dynamics/Motor_rotor_Dynamics/motor4/control_speed ==
  data: error output; prev_error input; u input; y output; int_u input; desired input; P parameter
function [error, y] = fcn(prev_error, u, int_u, desired, P)

%y = u;
if desired > 1000
    desired = 1000;
end

error = (desired-u);

Ts = P.Ts;

% kd = .2;
% kp = 10;
% ki = 5;

% kd = 0.05;
% kp = 1;
% ki = 1;

kd = P.kd_motor;
kp = P.kp_motor;
ki = P.ki_motor;

edot = ((error)-(prev_error))/Ts;

y = (kd*edot + kp*(error) + ki*int_u);

%saturate pwm at 2000
if abs(y) > 2000
    y = sign(y)*2000;
end

== matlab function quadABLwind/quadrotor/Reshape output ==
  data: state input; y output; euler input
function y = fcn(state, euler)

y = zeros(12,1);

y(1:6) = state(1:6);
y(7:9) = euler;

phi = euler(1);
theta = euler(2);
psi = euler(3);
Reuler = [1 sin(phi)*tan(theta) cos(phi)*tan(theta);
          0 cos(phi) -sin(phi);
          0 sin(phi)/cos(theta) cos(phi)/cos(theta)];


y(10:12) = Reuler*state(10:12);

== matlab function quadABLwind/quadrotor/Motor-Rotor_Dynamics/Motor_rotor_Dynamics/moments_to_motor_speeds ==
  data: u input; omega output; P parameter
function omega = fcn(u, P)

omega = u;
u(3) = -u(3);
%prevent negative F
if u(1)<0
    u(1)=0;
end
%prevent too high of a moment
for i=2:3
    if u(i)>.15*u(1)
        u(i)=.15*u(1);
    end
end

L = P.L;
k_t = P.k_t;
k_d = P.k_d;
offset = pi/4;

A = [k_t k_t k_t k_t;
    0 -L*k_t 0 L*k_t;
    L*k_t 0 -L*k_t 0;
    k_d -k_d k_d -k_d];

R = [1 0 0 0;
    0 cos(offset) -sin(offset) 0;
    0 sin(offset) cos(offset) 0;
    0 0 0 1];

omega_squared = pinv(A)*R*u;

for i=1:4
    if omega_squared(i) < 0
        omega_squared(i) = 0;
    end
end



omega = sqrt(omega_squared);

== matlab function quadABLwind/quadrotor/Motor-Rotor_Dynamics/Motor_rotor_Dynamics/motor1/control_speed ==
  data: error output; prev_error input; u input; y output; int_u input; desired input; P parameter
function [error, y] = fcn(prev_error, u, int_u, desired, P)

%y = u;
if desired > 1000
    desired = 1000;
end

error = (desired-u);

Ts = P.Ts;

% kd = .2;
% kp = 10;
% ki = 5;

% kd = 0.05;
% kp = 1;
% ki = 1;

kd = P.kd_motor;
kp = P.kp_motor;
ki = P.ki_motor;

edot = ((error)-(prev_error))/Ts;

y = (kd*edot + kp*(error) + ki*int_u);

%saturate pwm at 2000
if abs(y) > 2000
    y = sign(y)*2000;
end

== matlab function quadABLwind/quadrotor/Att Controller1 ==
  data: x input; u output; desired input; prev_x input; P parameter
function u = fcn(x, desired, prev_x, P)
%#codegen
% Reference: A Simple Attitude Control of Quadrotor Helicopter Based on
%Ziegler-Nichols Rules for Tuning PD Parameters

%ZeFang He and Long Zhao

u = zeros(4,1);
%timestep size
Ts = P.Ts;

L = P.L;  Ix = P.Ix;  Iy = P.Iy;  Iz = P.Iz; m = P.m; g = P.g;
b1 = 1/Ix;
b2 = 1/Iy;
b3 = 1/Iz;

a1 = (Iy-Iz)/Ix;
a3 = (Iz-Ix)/Iy;
a5 = (Ix-Iy)/Iz;

K2 = P.K2;
K3 = P.K3;
K4 = P.K4;

Kp2 = P.Kp2;
Kp3 = P.Kp3;
Kp4 = P.Kp4;

Kd2 = P.Kd2;
Kd3 = P.Kd3;
Kd4 = P.Kd4;


err2 = (desired(7) - x(7));
err3 = (desired(8) - x(8));
err4 = (desired(9) - x(9));
prev_err2 = (desired(7) - prev_x(7));
prev_err3 = (desired(8) - prev_x(8));
prev_err4 = (desired(9) - prev_x(9));

err_tot = [err2;err3;err4];
prev_err_tot = [prev_err2;prev_err3;prev_err4];

u(1) = (m*g + desired(3)*m)/(cos(x(7)) * cos(x(8)));
% u(2) = 1/b1*(K2*x(10)-a1*x(11)*x(12)) + Kp2*err2 + Kd2*(err2-prev_err2)/Ts;
% u(3) = 1/b2*(K3*x(11)-a3*x(10)*x(12)) + Kp3*err3 + Kd3*(err3-prev_err3)/Ts;
% u(4) = 1/b3*(K4*x(12)-a5*x(10)*x(11)) + Kp4*err4 + Kd4*(err4-prev_err4)/Ts;
u(2:4) = P.I*(K2*x(10:12)) + cross(x(10:12),P.I*x(10:12)) + Kp2*err_tot + Kd2*(err_tot-prev_err_tot)/Ts;

% u(1) = (m*g + desired(3)*m)/(cos(euler(1)) * cos(euler(2)));
% u(2) = 1/b1*(K2*x(10)-a1*x(11)*x(12)) + Kp2*err2 + Kd2*(err2-prev_err2)/Ts;
% u(3) = 1/b2*(K3*x(11)-a3*x(10)*x(12)) + Kp3*err3 + Kd3*(err3-prev_err3)/Ts;
% u(4) = 1/b3*(K4*x(12)-a5*x(10)*x(11)) + Kp4*err4 + Kd4*(err4-prev_err4)/Ts;

== matlab function quadABLwind/Position Control/Position Controller2 ==
  data: x input; prev_state input; sumError input; u input; y output; wind_and_Max_Vel input; P parameter
function y  = fcn(x, prev_state, sumError, u, wind_and_Max_Vel, P)
%#codegen
%PID controller tuned by hand

R2D = [cos(x(9)), -sin(x(9)); sin(x(9)), cos(x(9))];

% u = xyz, yaw
y = zeros(12,1);
Ts = P.Ts;
g = P.g;
m = P.m;

Cd=zeros(3,1);
Cd(1:3) = P.Cd1 + 0.9*exp(-0.6*(norm(wind_and_Max_Vel+x(4))-2));
for i=1:3
    if Cd(i) > 1.1
        Cd(i) = 1.1;
    end
end 

%control 7,8,9 for roll, pitch, yaw angles
u = -u;

x_error1 = (u(1) + x(1));
y_error1 = (u(2) + x(2));
%x_error = (u(1) + x(1));
%y_error = (u(2) + x(2));
z_error = u(3) + x(3);

%rotate to correct to roll, pitch
xerror2 = R2D*[x_error1; y_error1];
x_error = xerror2(1);
y_error = xerror2(2);

%previous errors
px_error1 = (u(1) + prev_state(1));
py_error1 = (u(2) + prev_state(2));
pz_error = u(3) + prev_state(3);

pxerror2 = R2D*[px_error1; py_error1];
px_error = pxerror2(1);
py_error = pxerror2(2);


vx_error1 = (u(4) + x(4));
vy_error1 = (u(5) + x(5));

vxerror2 = R2D*[vx_error1; vy_error1];
vx_error = vxerror2(1);
vy_error = vxerror2(2);

kp = P.kp;
kd = P.kd;
%ki currently set to zero.  Using PD control
ki = P.ki;


%PID controller for y, x, and yaw.  Sends roll/pitch angles to attitude
%controller
y(7) = (kp*y_error + kd*vy_error) + ki*sumError(2);
y(8) = (kp*x_error + kd*vx_error) + ki*sumError(1);


y(9) = -u(7);

k2 = P.k2;
kd2 = P.kd2;
ki2 = P.ki2;
%altitude control
y(3) = k2*z_error + kd2*(z_error - pz_error)/Ts + ki2*sumError(3);

% if abs(y(3))>6
%     y(3)=sign(y(3))*6;
% end

%ensure that the norm of velocity is correct since the pitch is hardcoded
if abs(wind_and_Max_Vel(3)) < abs(x(4))
    wind_and_Max_Vel(3) = x(4);
end

mag_V = wind_and_Max_Vel(1:2) + wind_and_Max_Vel(3:4);
mag_Combined = norm(mag_V); %airspeed magnitude

F_w = zeros(2,1);
F_w(1) = Cd(1) * mag_Combined^2;
F_w(2) = Cd(2) * mag_Combined^2;

%roll, pitch angles determined by desired y, x velocities and windspeed
max_Angle = zeros(1,2);
max_Angle(1) = 0.8;%atan2(F_w(2) * mag_V(2), m*g*mag_Combined);
max_Angle(2) = 0.8;%0.535;

if max_Angle(1) > 0.8
    max_Angle(1) = 0.8;
end

if y(7) > max_Angle(1)
    y(7) = max_Angle(1);

elseif y(7) < -max_Angle(1)
    y(7) = -max_Angle(1);
end
if y(8) > max_Angle(2)
    y(8) = max_Angle(2);
elseif y(8) < -max_Angle(2)
    y(8) = -max_Angle(2);
end

%set maximum total angle to 0.8 radians
% angleNorm = norm(y(7:8));
% if angleNorm > 0.8
%     y(7) = y(7)/(angleNorm)*(0.8);
%     y(8) = y(8)/(angleNorm)*(0.8);
% end

end

== matlab function quadABLwind/wind generation2/MATLAB Function1 ==
  data: trigger output; u input; time input; y output
function [trigger, y] = fcn(u, time)
%#codegen
y = u;

if mod(time, 0.1) == 0
    trigger = time;
else
    trigger = 0;
end

end

== matlab function quadABLwind/quadrotor/Motor-Rotor_Dynamics/Motor_rotor_Dynamics/motor_speed_to_moments ==
  data: u input; F output; P parameter
function F = fcn(u, P)

F = u;

L = P.L;
k_t = P.k_t;
k_d = P.k_d;
offset = pi/4;

A = [k_t k_t k_t k_t;
    0 -L*k_t 0 L*k_t;
    L*k_t 0 -L*k_t 0;
    k_d -k_d k_d -k_d];

R = [1 0 0 0;
    0 cos(offset) -sin(offset) 0;
    0 sin(offset) cos(offset) 0;
    0 0 0 1];

F = A*u.^2;
F = R*F;

F(2:3)=F(3:-1:2);

== matlab function quadABLwind/wind generation2/get_Wind/Send appropriate input ==
  data: state input; windspeed input; windspeedN input; starting_Point input; y output; time input
function y = fcn(state, windspeed, windspeedN, starting_Point, time)
%#codegen


if state(1) > 400-starting_Point(1)
    error = "Out of windfield, error"
    pause()
end

wind_t1 = 0;
wind_t2 = 0;
windN_t1 = 0;
windN_t2 = 0;
t1 = 0;

for i=1:6
    if time >= (i-1)*10 && time <= i*10
        wind_t1 = windspeed(((i-1)*32000+1):i*32000, :);
        wind_t2 = windspeed(((i)*32000):(i+1)*32000, :);
        windN_t1 = windspeedN(((i-1)*32000+1):i*32000, :);
        windN_t2 = windspeedN(((i)*32000):(i+1)*32000, :);
        t1 = (i-1)*10;
    end
end


%center state in windfield and normalize to 2 meter steps
adjusted_State = round((state(1:3) + starting_Point)/2);
adjusted_State(3) = adjusted_State(3) * 200;


new_Wind1 = wind_t1((adjusted_State(3)+adjusted_State(2)), adjusted_State(1));
new_Wind2 = wind_t2((adjusted_State(3)+adjusted_State(2)), adjusted_State(1));
interpolated_Wind = (new_Wind2 - new_Wind1)/10 * (time - t1) + new_Wind1;

new_WindN1 = windN_t1((adjusted_State(3)+adjusted_State(2)), adjusted_State(1));
new_WindN2 = windN_t2((adjusted_State(3)+adjusted_State(2)), adjusted_State(1));
interpolated_WindN = (new_WindN2 - new_WindN1)/10 * (time - t1) + new_WindN1;

y = [interpolated_WindN; interpolated_Wind; 0];
time


end
